simulink model "Week1problem2"  (R2020b)
settings: Solver=VariableStepAuto  StartTime=0.0  StopTime=10.0  RelTol=1e-3
model workspace (MAT data in the model file):
  b = 9000
  k1 = 12000
  k2 = 10000
  m1 = 1000
  m2 = 100
settings Model: Creator=Admin  LastModifiedBy=Admin

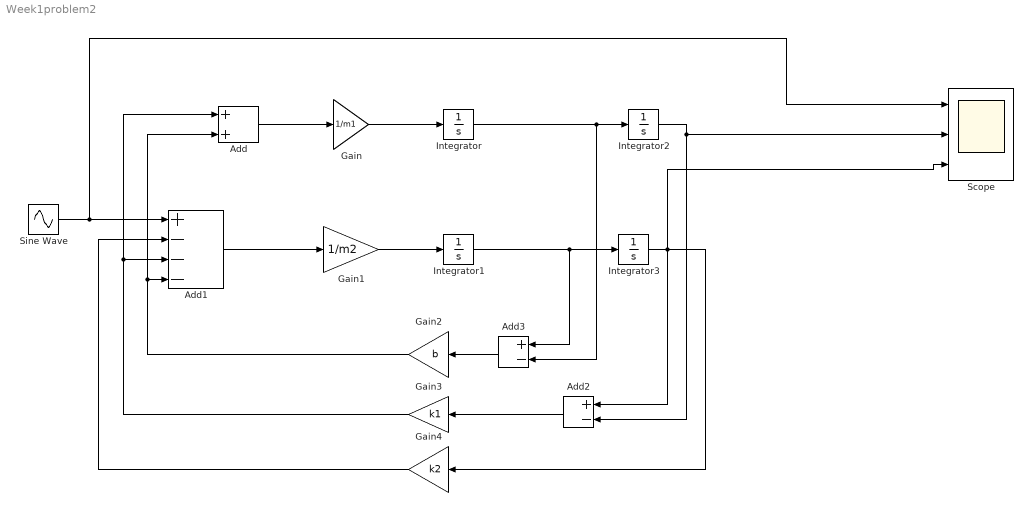
== system Week1problem2 ==
  Add : Sum
  Add1 : Sum  Inputs=+---
  Add2 : Sum  Inputs=+-
  Add3 : Sum  Inputs=+-
  Gain : Gain  Gain=1/m1
  Gain1 : Gain  Gain=1/m2
  Gain2 : Gain  Gain=b
  Gain3 : Gain  Gain=k1
  Gain4 : Gain  Gain=k2
  Integrator{,1..3} (4 alike) : Integrator
  Scope : Scope  NumInputPorts=3
  Sine Wave : Sin  Frequency=10  SampleTime=0
  wires:
  Sine Wave/1 -> Scope/1, Add1/1
  Add1/1 -> Gain1/1
  Gain1/1 -> Integrator1/1
  Integrator1/1 -> Add3/1, Integrator3/1
  Integrator/1 -> Integrator2/1, Add3/2
  Gain3/1 -> Add1/3, Add/1
  Gain2/1 -> Add1/4, Add/2
  Gain4/1 -> Add1/2
  Add3/1 -> Gain2/1
  Integrator2/1 -> Add2/2, Scope/2
  Integrator3/1 -> Gain4/1, Scope/3, Add2/1
  Add2/1 -> Gain3/1
  Add/1 -> Gain/1
  Gain/1 -> Integrator/1
